simulink model "Multi_Agent_Problem"  (R2022a)
settings: Solver=ode45  StartTime=0.0  StopTime=20  RelTol=1e-3
values from neighbouring files (symbols this model uses):
  B1_inv = B1_inv(:,2)    [Dynamic_Inversion.m]    (also in Linear_Model.mat = [0.0377096774194 0 -0.0377096774194 0])
  B2_inv = B2_inv(:,2)    [Dynamic_Inversion.m]    (also in Linear_Model.mat = [0 -0.0371290322581 0 0.0371290322581])
  B3_inv = B3_inv(:,1)    [Dynamic_Inversion.m]    (also in Linear_Model.mat = [0.0031875 -0.0031875 0.0031875 -0.0031875])
  B4_inv = pinv(B4)    [Dynamic_Inversion.m]    (also in Linear_Model.mat = [-0.25 -0.25 -0.25 -0.25])
  eta = 1    [Properties_Quad.m]
  g = 9.8    [Properties_Quad.m]
  L = 0.155    [Properties_Quad.m]
  m = 4    [Controller_LQR.m]    (also in Properties_Quad.m = 1)
  mass = 0.9    [Properties_Quad.m]
  r = [ones(1,length(t))]    [Hinf_Controller_Create.m]    (also in Properties_Quad.m = 1.5)
  u_e = zeros(4,1)    [Controller_LQR.m]    (also in Dynamic_Inversion.m; Linear_Model.mat = [2.45 2.45 2.45 2.45])
  w1_in = 4    [Dynamic_Inversion.m]    (also in Linear_Model.mat)
  w1_out = 1    [Dynamic_Inversion.m]    (also in Linear_Model.mat)
  w2_in = 4    [Dynamic_Inversion.m]    (also in Linear_Model.mat)
  w2_out = 1    [Dynamic_Inversion.m]    (also in Linear_Model.mat)
  w3_in = 4    [Dynamic_Inversion.m]    (also in Linear_Model.mat)
  w4_in = 3    [Dynamic_Inversion.m]    (also in Linear_Model.mat)
  zeta1_in = 0.7    [Dynamic_Inversion.m]    (also in Linear_Model.mat)
  zeta1_out = 0.7    [Dynamic_Inversion.m]    (also in Linear_Model.mat)
  zeta2_in = 0.7    [Dynamic_Inversion.m]    (also in Linear_Model.mat)
  zeta2_out = 0.7    [Dynamic_Inversion.m]    (also in Linear_Model.mat)
  zeta3_in = 0.7    [Dynamic_Inversion.m]    (also in Linear_Model.mat)
  zeta4_in = 0.7    [Dynamic_Inversion.m]    (also in Linear_Model.mat)
undefined symbols (not defined in the file or in its folder): magnitude
libraries: aerolibutil x4, rllib x3, shared6dof x3
(part 2 of 2)

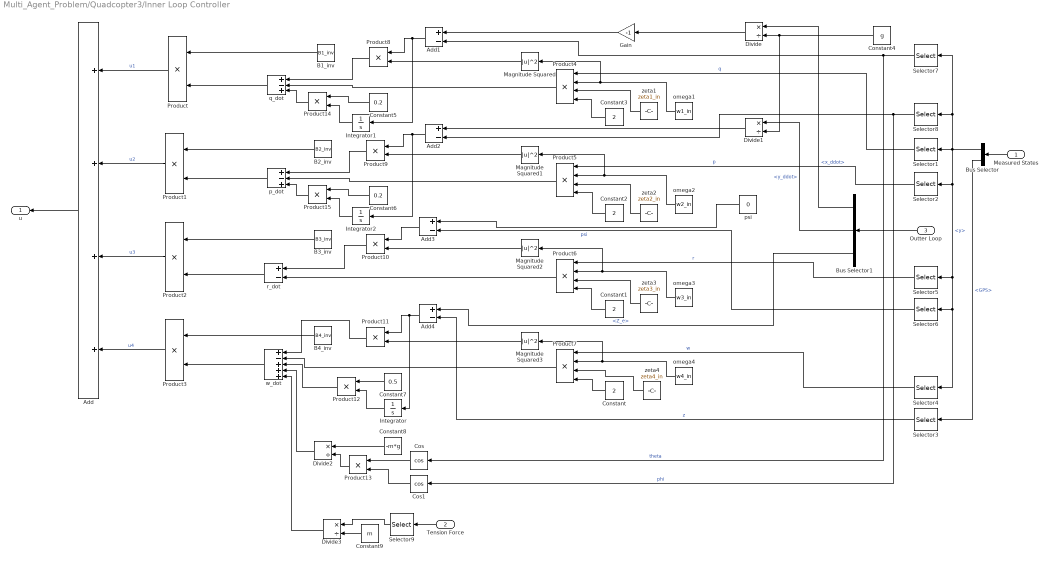
== system Multi_Agent_Problem/Quadcopter3/Inner Loop Controller ==
  Measured States : Inport
  Tension Force : Inport  Port=2
  Outter Loop : Inport  Port=3
  Add : Sum  Inputs=++++
  Add{1..4} (4 alike) : Sum  Inputs=+-
  B1_inv : Constant  Value=B1_inv
  B2_inv : Constant  Value=B2_inv
  B3_inv : Constant  Value=B3_inv
  B4_inv : Constant  Value=B4_inv
  Bus Selector : BusSelector  OutputSignals=y,GPS
  Bus Selector1 : BusSelector  OutputSignals=x_ddot,y_ddot,Z_e
  Constant{,1..3} (4 alike) : Constant  Value=2
  Constant4 : Constant  Value=g
  Constant5 : Constant  Value=0.2
  Constant6 : Constant  Value=0.2
  Constant7 : Constant  Value=0.5
  Constant8 : Constant  Value=-m*g
  Constant9 : Constant  Value=m
  Cos : Trigonometry  Operator=cos
  Cos1 : Trigonometry  Operator=cos
  Divide{,1..3} (4 alike) : Product  Inputs=*/
  Gain : Gain  Gain=-1
  Integrator : Integrator
  Integrator1 : Integrator
  Integrator2 : Integrator
  Magnitude Squared{,1..3} (4 alike) : Math  Operator=magnitude^2
  Product{,1..3,8..15} (12 alike) : Product
  Product{4..7} (4 alike) : Product  Inputs=4
  Selector1 : Selector  InputPortWidth=9  IndexOptions=Index vector (dialog)  Indices=5  OutputSizes=1
  Selector2 : Selector  InputPortWidth=9  IndexOptions=Index vector (dialog)  Indices=4  OutputSizes=1
  Selector3 : Selector  InputPortWidth=3  IndexOptions=Index vector (dialog)  Indices=3  OutputSizes=1
  Selector4 : Selector  InputPortWidth=9  IndexOptions=Index vector (dialog)  Indices=3  OutputSizes=1
  Selector5 : Selector  InputPortWidth=9  IndexOptions=Index vector (dialog)  Indices=6  OutputSizes=1
  Selector6 : Selector  InputPortWidth=9  IndexOptions=Index vector (dialog)  Indices=9  OutputSizes=1
  Selector7 : Selector  InputPortWidth=9  IndexOptions=Index vector (dialog)  Indices=8  OutputSizes=1
  Selector8 : Selector  InputPortWidth=9  IndexOptions=Index vector (dialog)  Indices=7  OutputSizes=1
  Selector9 : Selector  InputPortWidth=3  IndexOptions=Index vector (dialog)  Indices=3  OutputSizes=1
  omega1 : Constant  Value=w1_in
  omega2 : Constant  Value=w2_in
  omega3 : Constant  Value=w3_in
  omega4 : Constant  Value=w4_in
  p_dot : Sum  Inputs=+-+
  psi : Constant  Value=0
  q_dot : Sum  Inputs=+-+
  r_dot : Sum  Inputs=+-
  w_dot : Sum  Inputs=+-+++
  zeta1 : Constant  Value=zeta1_in
  zeta2 : Constant  Value=zeta2_in
  zeta3 : Constant  Value=zeta3_in
  zeta4 : Constant  Value=zeta4_in
  u : Outport
  wires:
  Add/1 -> u/1
  Product/1 -> Add/1  "u1"
  Product1/1 -> Add/2  "u2"
  Product2/1 -> Add/3  "u3"
  Product3/1 -> Add/4  "u4"
  B1_inv/1 -> Product/1
  B2_inv/1 -> Product1/1
  B3_inv/1 -> Product2/1
  B4_inv/1 -> Product3/1
  q_dot/1 -> Product/2
  p_dot/1 -> Product1/2
  r_dot/1 -> Product2/2
  w_dot/1 -> Product3/2
  Product8/1 -> q_dot/1
  Product9/1 -> p_dot/1
  Product10/1 -> r_dot/1
  Product11/1 -> w_dot/1
  Product4/1 -> q_dot/2
  Product5/1 -> p_dot/2
  Product6/1 -> r_dot/2
  Product7/1 -> w_dot/2
  Magnitude Squared/1 -> Product8/2
  Magnitude Squared1/1 -> Product9/2
  Magnitude Squared2/1 -> Product10/2
  Magnitude Squared3/1 -> Product11/2
  Constant/1 -> Product7/4
  Constant1/1 -> Product6/4
  Constant2/1 -> Product5/4
  Constant3/1 -> Product4/4
  zeta1/1 -> Product4/3
  zeta2/1 -> Product5/3
  zeta3/1 -> Product6/3
  omega1/1 -> Magnitude Squared/1, Product4/2
  omega2/1 -> Magnitude Squared1/1, Product5/2
  omega3/1 -> Magnitude Squared2/1, Product6/2
  omega4/1 -> Magnitude Squared3/1, Product7/2
  Measured States/1 -> Bus Selector/1
  Selector1/1 -> Product4/1  "q"
  Selector2/1 -> Product5/1  "p"
  Selector5/1 -> Product6/1  "r"
  Selector4/1 -> Product7/1  "w"
  zeta4/1 -> Product7/3
  Add3/1 -> Product10/1
  Add4/1 -> Integrator/1, Product11/1
  Outter Loop/1 -> Bus Selector1/1
  Bus Selector1/1 -> Divide/1  "<x_ddot>"
  Bus Selector1/2 -> Divide1/1  "<y_ddot>"
  psi/1 -> Add3/1
  Bus Selector1/3 -> Add4/1  "<Z_e>"
  Bus Selector/1 -> Selector5/1, Selector6/1, Selector4/1, Selector2/1, Selector1/1, Selector8/1, Selector7/1  "<y>"
  Divide/1 -> Gain/1
  Constant4/1 -> Divide1/2, Divide/2
  Bus Selector/2 -> Selector3/1  "<GPS>"
  Selector3/1 -> Add4/2  "z"
  Selector6/1 -> Add3/2  "psi"
  Selector8/1 -> Cos1/1, Add2/2  "phi"
  Selector7/1 -> Cos/1, Add1/2  "theta"
  Gain/1 -> Add1/1
  Divide1/1 -> Add2/1
  Constant7/1 -> Product12/1
  Integrator/1 -> Product12/2
  Product12/1 -> w_dot/3
  Cos/1 -> Product13/1
  Cos1/1 -> Product13/2
  Constant8/1 -> Divide2/1
  Product13/1 -> Divide2/2
  Divide2/1 -> w_dot/4
  Integrator1/1 -> Product14/2
  Add1/1 -> Integrator1/1, Product8/1
  Product14/1 -> q_dot/3
  Constant5/1 -> Product14/1
  Constant6/1 -> Product15/1
  Product15/1 -> p_dot/3
  Add2/1 -> Integrator2/1, Product9/1
  Integrator2/1 -> Product15/2
  Divide3/1 -> w_dot/5
  Constant9/1 -> Divide3/2
  Selector9/1 -> Divide3/1
  Tension Force/1 -> Selector9/1

== system Multi_Agent_Problem/Quadcopter3/Mission Planner ==
  GPS : Inport
  states : Inport  Port=2
  Mass_L : Inport  Port=3
  Build Observation Vector : Subsystem
  Bus Creator : BusCreator  Inputs=3
  Bus Creator1 : BusCreator  Inputs=3
  Bus Selector : BusSelector  OutputSignals=GPS1,GPS2,GPS3
  Constant : Constant  Value=4
  Constant2 : Constant  Value=-1.5
  Constant3 : Constant  Value=(1 + sqrt(1.25))
  Demux : Demux  Outputs=3
  Find Reward : MATLAB Function  TreatAsAtomicUnit=on
  RL Agent3 : rllib/RL Agent  Agent=agent3  ExternalActionAsInput=off  ProvideLastAction=off  ProvideCumRwd=off  TreatAsDirectFeedthrough=on  UseStrictObservationDataTypes=off
  Terminator : Terminator
  Mission Planner : Outport
  wires:
  Constant/1 -> Bus Creator/1  "x_e"
  Constant2/1 -> Bus Creator/2  "y_e"
  Constant3/1 -> Bus Creator/3  "h_e"
  GPS/1 -> Bus Selector/1, Build Observation Vector/2(GPS)
  Find Reward/1(reward) -> RL Agent3/2
  Find Reward/2(isdone) -> RL Agent3/3
  states/1 -> Build Observation Vector/1(states)
  Build Observation Vector/1(Obsv) -> RL Agent3/1
  RL Agent3/1 -> Demux/1
  Demux/1 -> Bus Creator1/1  "x_e"
  Demux/2 -> Bus Creator1/2  "y_e"
  Demux/3 -> Bus Creator1/3  "z_e"
  Bus Creator1/1 -> Terminator/1
  Bus Selector/1 -> Find Reward/1(GPS1)  "<GPS1>"
  Bus Selector/2 -> Find Reward/2(GPS2)  "<GPS2>"
  Bus Selector/3 -> Find Reward/3(GPS3)  "<GPS3>"
  Mass_L/1 -> Build Observation Vector/3(mass_l), Find Reward/4(GPS4)
  Bus Creator/1 -> Mission Planner/1

== system Multi_Agent_Problem/Quadcopter3/Nonlinear System ==
  Resulting Force : Inport
  u : Inport  Port=2
  6DOF (Euler Angles) : shared6dof/6DOF (Euler Angles)  units=Metric (MKS)  mtype=Fixed  rep=Euler Angles  xme_0=init_3.pos_e  Vm_0=init_3.vel_b  eul_0=init_3.Euler  pm_0=init_3.rotation_rates_b  mass_0=m  mass_e=0.5  mass_f=2.0  inertia=I  inertia_e=eye(3)  inertia_f=2*eye(3)  k_quat=1.0  vre_flag=on  abi_flag=off  aMode=0  xme_statename=''  Vm_statename=''  eul_statename=''  quat_statename=''  pm_statename=''  mass_statename=''
      settings: SourceProductBaseCode=AE,PW,DR,MT,VE
  Add : Sum
  Matrix Concatenate : Concatenate  NumInputs=3  ConcatenateDimension=2
  Product : Product  Multiplication=Matrix(*)
  Solve for Forces : Subsystem
  Solve for Moments : Subsystem
  Terminator1 : Terminator
  Terminator2 : Terminator
  Terminator3 : Terminator
  X_e : Outport
  x : Outport  Port=2
  E2B : Outport  Port=3
  wires:
  6DOF (Euler Angles)/8 -> Terminator3/1
  6DOF (Euler Angles)/1 -> Matrix Concatenate/1
  6DOF (Euler Angles)/7 -> Terminator2/1
  u/1 -> Solve for Moments/1(u), Solve for Forces/2(u)
  6DOF (Euler Angles)/6 -> Matrix Concatenate/2
  6DOF (Euler Angles)/3 -> Matrix Concatenate/3
  6DOF (Euler Angles)/5 -> Terminator1/1
  Solve for Forces/1(Forces) -> Add/2
  Solve for Moments/1(Moments) -> 6DOF (Euler Angles)/2
  6DOF (Euler Angles)/2 -> X_e/1
  Matrix Concatenate/1 -> x/1
  Resulting Force/1 -> Product/2
  Add/1 -> 6DOF (Euler Angles)/1
  6DOF (Euler Angles)/4 -> Product/1, E2B/1, Solve for Forces/1(E2B)
  Product/1 -> Add/1

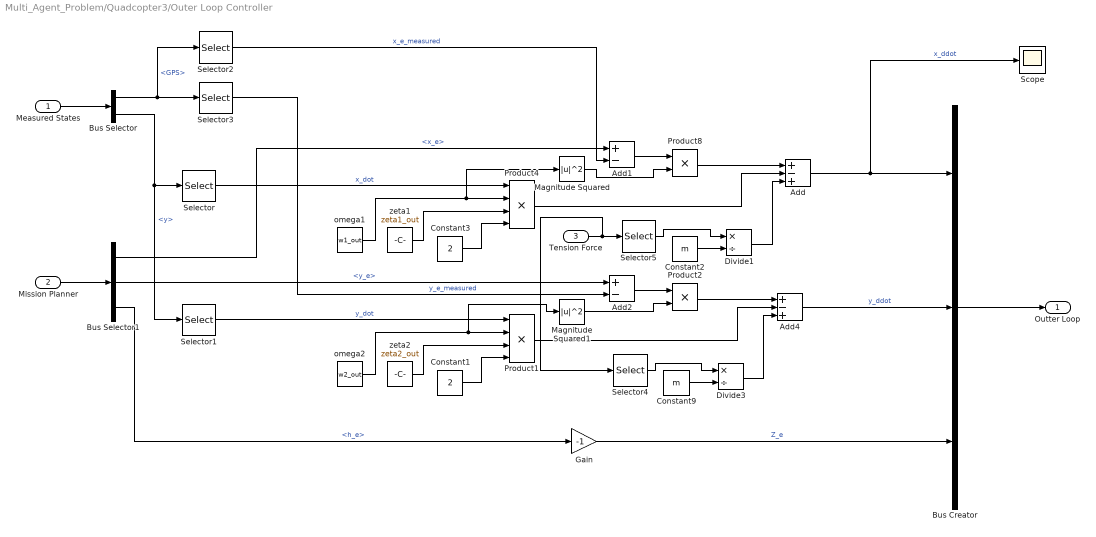
== system Multi_Agent_Problem/Quadcopter3/Outer Loop Controller ==
  Measured States : Inport
  Mission Planner : Inport  Port=2
  Tension Force : Inport  Port=3
  Add : Sum  Inputs=+-+
  Add1 : Sum  Inputs=+-
  Add2 : Sum  Inputs=+-
  Add4 : Sum  Inputs=+-+
  Bus Creator : BusCreator  Inputs=3
  Bus Selector : BusSelector  OutputSignals=GPS,y
  Bus Selector1 : BusSelector  OutputSignals=x_e,y_e,h_e
  Constant1 : Constant  Value=2
  Constant2 : Constant  Value=m
  Constant3 : Constant  Value=2
  Constant9 : Constant  Value=m
  Divide1 : Product  Inputs=*/
  Divide3 : Product  Inputs=*/
  Gain : Gain  Gain=-1
  Magnitude Squared : Math  Operator=magnitude^2
  Magnitude Squared1 : Math  Operator=magnitude^2
  Product1 : Product  Inputs=4
  Product2 : Product
  Product4 : Product  Inputs=4
  Product8 : Product
  Scope : Scope
  Selector : Selector  InputPortWidth=9  IndexOptions=Index vector (dialog)  Indices=1  OutputSizes=1
  Selector1 : Selector  InputPortWidth=9  IndexOptions=Index vector (dialog)  Indices=2  OutputSizes=1
  Selector2 : Selector  InputPortWidth=3  IndexOptions=Index vector (dialog)  Indices=1  OutputSizes=1
  Selector3 : Selector  InputPortWidth=3  IndexOptions=Index vector (dialog)  Indices=2  OutputSizes=1
  Selector4 : Selector  InputPortWidth=3  IndexOptions=Index vector (dialog)  Indices=2  OutputSizes=1
  Selector5 : Selector  InputPortWidth=3  IndexOptions=Index vector (dialog)  Indices=1  OutputSizes=1
  omega1 : Constant  Value=w1_out
  omega2 : Constant  Value=w2_out
  zeta1 : Constant  Value=zeta1_out
  zeta2 : Constant  Value=zeta2_out
  Outter Loop : Outport
  wires:
  Measured States/1 -> Bus Selector/1
  Selector/1 -> Product4/1  "x_dot"
  Product4/1 -> Add/2
  omega1/1 -> Magnitude Squared/1, Product4/2
  Bus Selector1/1 -> Add1/1  "<x_e>"
  Constant3/1 -> Product4/4
  Add1/1 -> Product8/1
  Add/1 -> Scope/1, Bus Creator/1  "x_ddot"
  zeta1/1 -> Product4/3
  Magnitude Squared/1 -> Product8/2
  Bus Creator/1 -> Outter Loop/1
  Mission Planner/1 -> Bus Selector1/1
  Bus Selector1/2 -> Add2/1  "<y_e>"
  Bus Selector/1 -> Selector3/1, Selector2/1  "<GPS>"
  Bus Selector/2 -> Selector1/1, Selector/1  "<y>"
  Selector2/1 -> Add1/2  "x_e_measured"
  Selector3/1 -> Add2/2  "y_e_measured"
  Magnitude Squared1/1 -> Product2/2
  zeta2/1 -> Product1/3
  Add4/1 -> Bus Creator/2  "y_ddot"
  Add2/1 -> Product2/1
  Constant1/1 -> Product1/4
  omega2/1 -> Magnitude Squared1/1, Product1/2
  Product1/1 -> Add4/2
  Product8/1 -> Add/1
  Product2/1 -> Add4/1
  Selector1/1 -> Product1/1  "y_dot"
  Bus Selector1/3 -> Gain/1  "<h_e>"
  Gain/1 -> Bus Creator/3  "Z_e"
  Divide3/1 -> Add4/3
  Constant9/1 -> Divide3/2
  Selector4/1 -> Divide3/1
  Divide1/1 -> Add/3
  Constant2/1 -> Divide1/2
  Selector5/1 -> Divide1/1
  Tension Force/1 -> Selector4/1, Selector5/1

== system Multi_Agent_Problem/Quadcopter3/Sensors ==
  X_e : Inport
  States : Inport  Port=2
  Bus Creator : BusCreator  Inputs=2
  Measured States : Outport
  wires:
  States/1 -> Bus Creator/2  "y"
  Bus Creator/1 -> Measured States/1
  X_e/1 -> Bus Creator/1  "GPS"

== system Multi_Agent_Problem/Quadcopter1/Mission Planner/Build Observation Vector ==
  states : Inport
  GPS : Inport  Port=2
  mass_l : Inport  Port=3
  Bus Selector : BusSelector  OutputSignals=y1,y2,y3
  Bus Selector2 : BusSelector  OutputSignals=GPS1,GPS2,GPS3
  Mux2 : Mux  Inputs=6
  Subtract : Sum  Inputs=+-
  Subtract1 : Sum  Inputs=+-
  Subtract2 : Sum  Inputs=+-
  Obsv : Outport
  wires:
  Bus Selector/1 -> Mux2/1  "<y1>"
  GPS/1 -> Bus Selector2/1
  states/1 -> Bus Selector/1
  Mux2/1 -> Obsv/1
  Bus Selector/2 -> Mux2/3  "<y2>"
  Bus Selector2/3 -> Subtract2/1  "<GPS3>"
  Bus Selector2/2 -> Subtract1/1  "<GPS2>"
  Bus Selector/3 -> Mux2/5  "<y3>"
  Subtract/1 -> Mux2/2
  Subtract1/1 -> Mux2/4
  Subtract2/1 -> Mux2/6
  Bus Selector2/1 -> Subtract/1  "<GPS1>"
  mass_l/1 -> Subtract2/2, Subtract1/2, Subtract/2

== system Multi_Agent_Problem/Quadcopter1/Nonlinear System/Solve for Forces ==
  E2B : Inport
  u : Inport  Port=2
  Add : Sum
  Constant : Constant  Value=-[0,0,1]
  Constant1 : Constant  Value=[0,0,1]
  Display : Display
  Display1 : Display
  Display2 : Display
  Force Gravity : Constant  Value=m*g
  Product : Product
  Product1 : Product
  Product2 : Product  Multiplication=Matrix(*)
  Sum of Elements : Sum  Inputs=+
  Forces : Outport
  wires:
  Product1/1 -> Product2/2
  Product2/1 -> Add/2
  Force Gravity/1 -> Product1/2
  Product/1 -> Display2/1, Add/1
  Constant1/1 -> Product1/1
  Constant/1 -> Product/2
  Sum of Elements/1 -> Product/1
  Add/1 -> Display/1, Forces/1
  u/1 -> Sum of Elements/1
  E2B/1 -> Display1/1, Product2/1

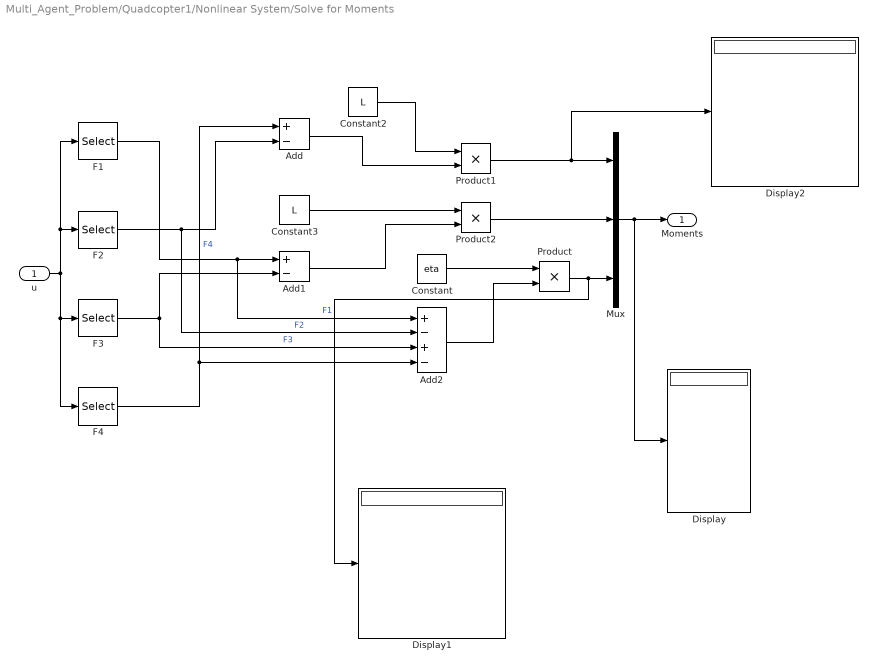
== system Multi_Agent_Problem/Quadcopter1/Nonlinear System/Solve for Moments ==
  u : Inport
  Add : Sum  Inputs=+-
  Add1 : Sum  Inputs=+-
  Add2 : Sum  Inputs=+-+-
  Constant : Constant  Value=eta
  Constant2 : Constant  Value=L
  Constant3 : Constant  Value=L
  Display : Display
  Display1 : Display
  Display2 : Display
  F1 : Selector  InputPortWidth=4  IndexOptions=Index vector (dialog)  Indices=1  OutputSizes=1
  F2 : Selector  InputPortWidth=4  IndexOptions=Index vector (dialog)  Indices=2  OutputSizes=1
  F3 : Selector  InputPortWidth=4  IndexOptions=Index vector (dialog)  Indices=3  OutputSizes=1
  F4 : Selector  InputPortWidth=4  IndexOptions=Index vector (dialog)  Indices=4  OutputSizes=1
  Mux : Mux  Inputs=3
  Product : Product
  Product1 : Product
  Product2 : Product
  Moments : Outport
  wires:
  Mux/1 -> Display/1, Moments/1
  u/1 -> F1/1, F2/1, F4/1, F3/1
  F2/1 -> Add2/2, Add/2  "F2"
  F3/1 -> Add2/3, Add1/2  "F3"
  F4/1 -> Add2/4, Add/1  "F4"
  Constant/1 -> Product/1
  Constant2/1 -> Product1/1
  Product1/1 -> Display2/1, Mux/1
  Product2/1 -> Mux/2
  Constant3/1 -> Product2/1
  Add/1 -> Product1/2
  Add1/1 -> Product2/2
  F1/1 -> Add2/1, Add1/1  "F1"
  Product/1 -> Display1/1, Mux/3
  Add2/1 -> Product/2

== system Multi_Agent_Problem/Quadcopter2/Mission Planner/Build Observation Vector ==
  states : Inport
  GPS : Inport  Port=2
  mass_l : Inport  Port=3
  Bus Selector : BusSelector  OutputSignals=y1,y2,y3
  Bus Selector2 : BusSelector  OutputSignals=GPS1,GPS2,GPS3
  Mux2 : Mux  Inputs=6
  Subtract : Sum  Inputs=+-
  Subtract1 : Sum  Inputs=+-
  Subtract2 : Sum  Inputs=+-
  Obsv : Outport
  wires:
  Bus Selector2/1 -> Subtract/1  "<GPS1>"
  Subtract2/1 -> Mux2/6
  Subtract1/1 -> Mux2/4
  Subtract/1 -> Mux2/2
  Bus Selector/3 -> Mux2/5  "<y3>"
  Bus Selector2/2 -> Subtract1/1  "<GPS2>"
  Bus Selector2/3 -> Subtract2/1  "<GPS3>"
  Bus Selector/2 -> Mux2/3  "<y2>"
  Mux2/1 -> Obsv/1
  states/1 -> Bus Selector/1
  GPS/1 -> Bus Selector2/1
  Bus Selector/1 -> Mux2/1  "<y1>"
  mass_l/1 -> Subtract2/2, Subtract1/2, Subtract/2

== system Multi_Agent_Problem/Quadcopter2/Nonlinear System/Solve for Forces ==
  E2B : Inport
  u : Inport  Port=2
  Add : Sum
  Constant : Constant  Value=-[0,0,1]
  Constant1 : Constant  Value=[0,0,1]
  Display : Display
  Display1 : Display
  Display2 : Display
  Force Gravity : Constant  Value=m*g
  Product : Product
  Product1 : Product
  Product2 : Product  Multiplication=Matrix(*)
  Sum of Elements : Sum  Inputs=+
  Forces : Outport
  wires:
  E2B/1 -> Product2/1, Display1/1
  u/1 -> Sum of Elements/1
  Add/1 -> Forces/1, Display/1
  Sum of Elements/1 -> Product/1
  Constant/1 -> Product/2
  Constant1/1 -> Product1/1
  Product/1 -> Add/1, Display2/1
  Force Gravity/1 -> Product1/2
  Product2/1 -> Add/2
  Product1/1 -> Product2/2

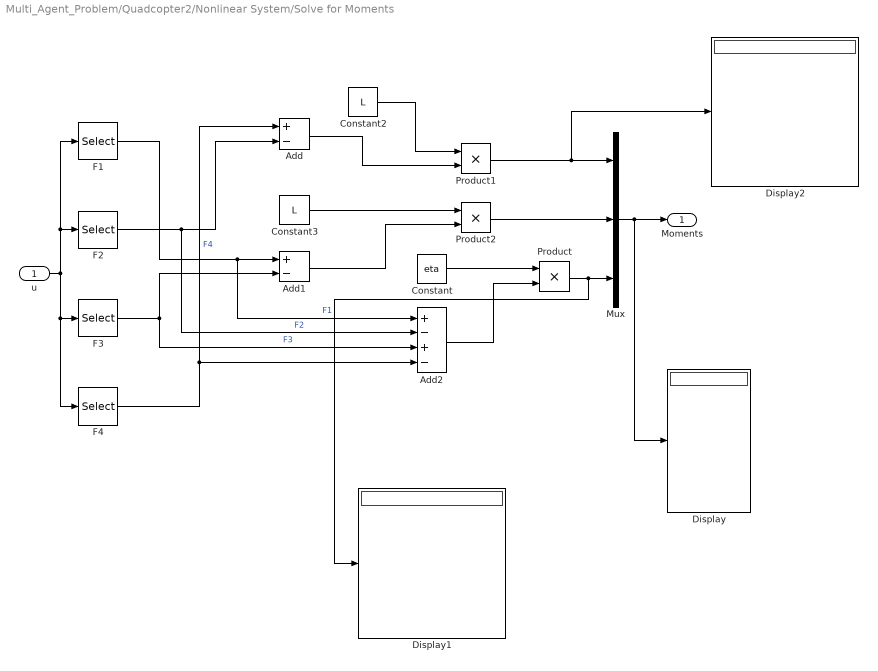
== system Multi_Agent_Problem/Quadcopter2/Nonlinear System/Solve for Moments ==
  u : Inport
  Add : Sum  Inputs=+-
  Add1 : Sum  Inputs=+-
  Add2 : Sum  Inputs=+-+-
  Constant : Constant  Value=eta
  Constant2 : Constant  Value=L
  Constant3 : Constant  Value=L
  Display : Display
  Display1 : Display
  Display2 : Display
  F1 : Selector  InputPortWidth=4  IndexOptions=Index vector (dialog)  Indices=1  OutputSizes=1
  F2 : Selector  InputPortWidth=4  IndexOptions=Index vector (dialog)  Indices=2  OutputSizes=1
  F3 : Selector  InputPortWidth=4  IndexOptions=Index vector (dialog)  Indices=3  OutputSizes=1
  F4 : Selector  InputPortWidth=4  IndexOptions=Index vector (dialog)  Indices=4  OutputSizes=1
  Mux : Mux  Inputs=3
  Product : Product
  Product1 : Product
  Product2 : Product
  Moments : Outport
  wires:
  Add2/1 -> Product/2
  Product/1 -> Mux/3, Display1/1
  F1/1 -> Add1/1, Add2/1  "F1"
  Add1/1 -> Product2/2
  Add/1 -> Product1/2
  Constant3/1 -> Product2/1
  Product2/1 -> Mux/2
  Product1/1 -> Mux/1, Display2/1
  Constant2/1 -> Product1/1
  Constant/1 -> Product/1
  F4/1 -> Add/1, Add2/4  "F4"
  F3/1 -> Add1/2, Add2/3  "F3"
  F2/1 -> Add/2, Add2/2  "F2"
  u/1 -> F3/1, F4/1, F2/1, F1/1
  Mux/1 -> Moments/1, Display/1

== system Multi_Agent_Problem/Quadcopter3/Mission Planner/Build Observation Vector ==
  states : Inport
  GPS : Inport  Port=2
  mass_l : Inport  Port=3
  Bus Selector : BusSelector  OutputSignals=y1,y2,y3
  Bus Selector2 : BusSelector  OutputSignals=GPS1,GPS2,GPS3
  Mux2 : Mux  Inputs=6
  Subtract : Sum  Inputs=+-
  Subtract1 : Sum  Inputs=+-
  Subtract2 : Sum  Inputs=+-
  Obsv : Outport
  wires:
  Bus Selector/1 -> Mux2/1  "<y1>"
  GPS/1 -> Bus Selector2/1
  states/1 -> Bus Selector/1
  Mux2/1 -> Obsv/1
  Bus Selector/2 -> Mux2/3  "<y2>"
  Bus Selector2/3 -> Subtract2/1  "<GPS3>"
  Bus Selector2/2 -> Subtract1/1  "<GPS2>"
  Bus Selector/3 -> Mux2/5  "<y3>"
  Subtract/1 -> Mux2/2
  Subtract1/1 -> Mux2/4
  Subtract2/1 -> Mux2/6
  Bus Selector2/1 -> Subtract/1  "<GPS1>"
  mass_l/1 -> Subtract1/2, Subtract/2, Subtract2/2

== system Multi_Agent_Problem/Quadcopter3/Nonlinear System/Solve for Forces ==
  E2B : Inport
  u : Inport  Port=2
  Add : Sum
  Constant : Constant  Value=-[0,0,1]
  Constant1 : Constant  Value=[0,0,1]
  Display : Display
  Display1 : Display
  Display2 : Display
  Force Gravity : Constant  Value=m*g
  Product : Product
  Product1 : Product
  Product2 : Product  Multiplication=Matrix(*)
  Sum of Elements : Sum  Inputs=+
  Forces : Outport
  wires:
  Product1/1 -> Product2/2
  Product2/1 -> Add/2
  Force Gravity/1 -> Product1/2
  Product/1 -> Display2/1, Add/1
  Constant1/1 -> Product1/1
  Constant/1 -> Product/2
  Sum of Elements/1 -> Product/1
  Add/1 -> Display/1, Forces/1
  u/1 -> Sum of Elements/1
  E2B/1 -> Display1/1, Product2/1

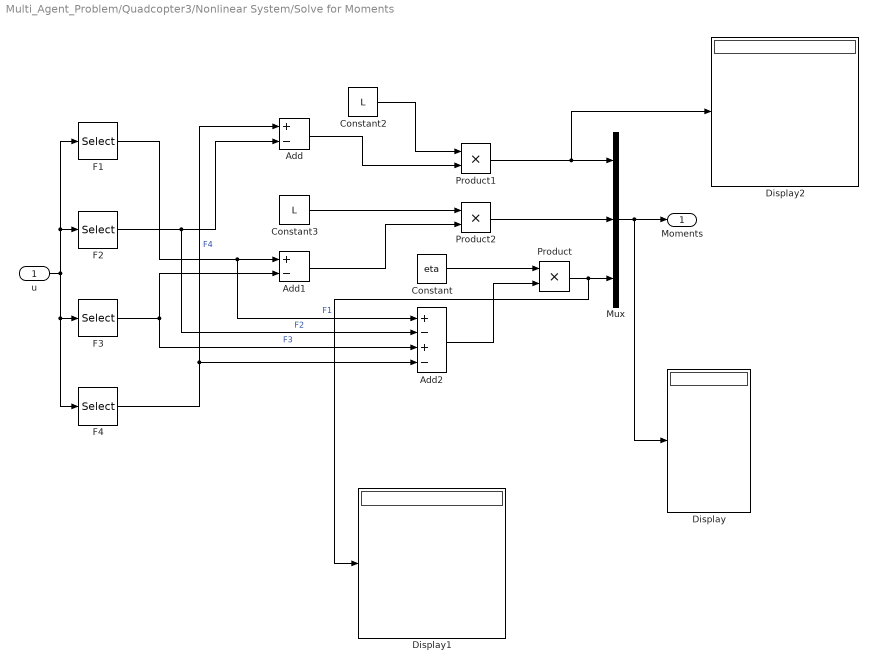
== system Multi_Agent_Problem/Quadcopter3/Nonlinear System/Solve for Moments ==
  u : Inport
  Add : Sum  Inputs=+-
  Add1 : Sum  Inputs=+-
  Add2 : Sum  Inputs=+-+-
  Constant : Constant  Value=eta
  Constant2 : Constant  Value=L
  Constant3 : Constant  Value=L
  Display : Display
  Display1 : Display
  Display2 : Display
  F1 : Selector  InputPortWidth=4  IndexOptions=Index vector (dialog)  Indices=1  OutputSizes=1
  F2 : Selector  InputPortWidth=4  IndexOptions=Index vector (dialog)  Indices=2  OutputSizes=1
  F3 : Selector  InputPortWidth=4  IndexOptions=Index vector (dialog)  Indices=3  OutputSizes=1
  F4 : Selector  InputPortWidth=4  IndexOptions=Index vector (dialog)  Indices=4  OutputSizes=1
  Mux : Mux  Inputs=3
  Product : Product
  Product1 : Product
  Product2 : Product
  Moments : Outport
  wires:
  Mux/1 -> Display/1, Moments/1
  u/1 -> F1/1, F2/1, F4/1, F3/1
  F2/1 -> Add2/2, Add/2  "F2"
  F3/1 -> Add2/3, Add1/2  "F3"
  F4/1 -> Add2/4, Add/1  "F4"
  Constant/1 -> Product/1
  Constant2/1 -> Product1/1
  Product1/1 -> Display2/1, Mux/1
  Product2/1 -> Mux/2
  Constant3/1 -> Product2/1
  Add/1 -> Product1/2
  Add1/1 -> Product2/2
  F1/1 -> Add2/1, Add1/1  "F1"
  Product/1 -> Display1/1, Mux/3
  Add2/1 -> Product/2

== matlab function Multi_Agent_Problem/Quadcopter2/Mission Planner/Find Reward ==
  data: GPS1 input; reward output; isdone output; GPS2 input; GPS3 input; GPS4 input
function [reward,isdone] = fcn(GPS1,GPS2,GPS3,GPS4)
    locations = [GPS1;GPS2;GPS3;GPS4];
    
    isdone = false;
    eps = 0.115; % Length of arm
    state = 0;
    for i = 1:3:4*3
        location = locations(i:i+2);
        % Maintain Bounds of the Box
        if location(1) < 0+eps
            s = -100;
            isdone = true;
        elseif location(1) > 6-eps
            s = -100;
            isdone = true;
        elseif location(2) > 0-eps
            s = -100;
            isdone = true;
        elseif location(3) > 0-eps
            s = -100;
            isdone = true;
        elseif location(3) < -6+eps
            s = -100;
            isdone = true;
        % Not through the doorway
        elseif location(2)<-2.5+eps && location(2)>-3.5-eps && (location(1)<2.2+eps || location(1)>3.8-eps)
            s = -100;
            isdone = true;
        elseif location(2)<-2.5+eps && location(2)>-3.5-eps && (location(3)>=0-eps || location(3)<-2.1+eps)
            s = -100;
            isdone = true;
        % On otherside of doorway
        elseif location(2) < -3.5-eps
            s = 1000;
        else
            s = 0;
        end
        state = state + s;
    end
    
    % Test for conlusions with other agents
    temp = [abs(GPS1-GPS2);abs(GPS1-GPS3);abs(GPS1-GPS4);...
        abs(GPS2-GPS3);abs(GPS2-GPS4);abs(GPS3-GPS4)];
    temp2 = sum(temp >= (2*eps));
    if temp2 > 0
        state = state - (100*temp2);
    end
    
    % End simulation because of reward
    if state > 4000
        isdone = true;
    end

    reward = state - 1;             % Adjust for taking an action -1
end

== matlab function Multi_Agent_Problem/Quadcopter1/Mission Planner/Find Reward ==
  data: GPS1 input; reward output; isdone output; GPS2 input; GPS3 input; GPS4 input
function [reward,isdone] = fcn(GPS1,GPS2,GPS3,GPS4)
    locations = [GPS1;GPS2;GPS3;GPS4];
    
    isdone = false;
    eps = 0.115; % Length of arm
    state = 0;
    for i = 1:3:4*3
        location = locations(i:i+2);
        % Maintain Bounds of the Box
        if location(1) < 0+eps
            s = -100;
            isdone = true;
        elseif location(1) > 6-eps
            s = -100;
            isdone = true;
        elseif location(2) > 0-eps
            s = -100;
            isdone = true;
        elseif location(3) > 0-eps
            s = -100;
            isdone = true;
        elseif location(3) < -6+eps
            s = -100;
            isdone = true;
        % Not through the doorway
        elseif location(2)<-2.5+eps && location(2)>-3.5-eps && (location(1)<2.2+eps || location(1)>3.8-eps)
            s = -100;
            isdone = true;
        elseif location(2)<-2.5+eps && location(2)>-3.5-eps && (location(3)>=0-eps || location(3)<-2.1+eps)
            s = -100;
            isdone = true;
        % On otherside of doorway
        elseif location(2) < -3.5-eps
            s = 1000;
        else
            s = 0;
        end
        state = state + s;
    end
    
    % Test for conlusions with other agents
    temp = [abs(GPS1-GPS2);abs(GPS1-GPS3);abs(GPS1-GPS4);...
        abs(GPS2-GPS3);abs(GPS2-GPS4);abs(GPS3-GPS4)];
    temp2 = sum(temp >= (2*eps));
    if temp2 > 0
        state = state - (100*temp2);
    end
    
    % End simulation because of reward
    if state > 4000
        isdone = true;
    end

    reward = state - 1;             % Adjust for taking an action -1
end

== matlab function Multi_Agent_Problem/Quadcopter3/Mission Planner/Find Reward ==
  data: GPS1 input; reward output; isdone output; GPS2 input; GPS3 input; GPS4 input
function [reward,isdone] = fcn(GPS1,GPS2,GPS3,GPS4)
    locations = [GPS1;GPS2;GPS3;GPS4];
    
    isdone = false;
    eps = 0.115; % Length of arm
    state = 0;
    for i = 1:3:4*3
        location = locations(i:i+2);
        % Maintain Bounds of the Box
        if location(1) < 0+eps
            s = -100;
            isdone = true;
        elseif location(1) > 6-eps
            s = -100;
            isdone = true;
        elseif location(2) > 0-eps
            s = -100;
            isdone = true;
        elseif location(3) > 0-eps
            s = -100;
            isdone = true;
        elseif location(3) < -6+eps
            s = -100;
            isdone = true;
        % Not through the doorway
        elseif location(2)<-2.5+eps && location(2)>-3.5-eps && (location(1)<2.2+eps || location(1)>3.8-eps)
            s = -100;
            isdone = true;
        elseif location(2)<-2.5+eps && location(2)>-3.5-eps && (location(3)>=0-eps || location(3)<-2.1+eps)
            s = -100;
            isdone = true;
        % On otherside of doorway
        elseif location(2) < -3.5-eps
            s = 1000;
        else
            s = 0;
        end
        state = state + s;
    end
    
    % Test for conlusions with other agents
    temp = [abs(GPS1-GPS2);abs(GPS1-GPS3);abs(GPS1-GPS4);...
        abs(GPS2-GPS3);abs(GPS2-GPS4);abs(GPS3-GPS4)];
    temp2 = sum(temp >= (2*eps));
    if temp2 > 0
        state = state - (100*temp2);
    end
    
    % End simulation because of reward
    if state > 4000
        isdone = true;
    end

    reward = state - 1;             % Adjust for taking an action -1
end

== matlab function Multi_Agent_Problem/Mass/Mass Location/Mass Location ==
  data: P1 input; mass_l output; P2 input; P3 input; r input
function mass_l = mass_location(P1,P2,P3,r)
% https://stackoverflow.com/questions/1406375/finding-intersection-points-between-3-spheres
    temp1 = P2-P1;
    temp2 = P3-P1;
    e_x = temp1/norm(temp1);                                                                  
    i = dot(e_x,temp2);                          
    temp3 = temp2 - i*e_x;
    e_y = temp3/norm(temp3);          
    e_z = cross(e_x,e_y);
    d = norm(P2-P1);
    j = dot(e_y,temp2);              
    x = (r*r - r*r + d*d) / (2*d);
    y = (r*r - r*r -2*i*x + i*i + j*j) / (2*j);
    temp4 = r*r - x*x - y*y;
    z = sqrt(temp4);
    p_12_a = P1 + x*e_x + y*e_y + z*e_z;
    %p_12_b = P1 + x*e_x + y*e_y - z*e_z;

    mass_l = p_12_a;
end
